simulink model "impedanceControl_ID_TUD"  (Simulink 7.9)
settings: Solver=FixedStepDiscrete  StartTime=0.0  StopTime=2000  FixedStep=Ts  RelTol=1e-3
InitFcn:
  | initialisation;
values from neighbouring files (symbols this model uses):
  A = 0*[20/180*pi;zeros(23,1);0/180*pi]    [initialisation.m]
  c = 0    [initialisation.m]
  D = diag(2*sqrt(20)*ones(1,25))    [initialisation.m]
  f = 0*1/100    (= 0)    [initialisation.m]
  P = diag(25*ones(1,25))    [initialisation.m]
  P_on = 0    [initialisation.m]
  s = 0*[10/180*pi/10;zeros(24,1)]    [initialisation.m]
  st = 0*[20/180*pi;0/180*pi;0/180*pi;0/180*pi;0/180*pi;zeros(20,1)]    [initialisation.m]
  tau_p = [torso_pitch; torso_roll; torso_yaw; left_shoulder_pitch; left_shoulder_roll; left_shoulder_yaw; left_elbow; left_wrist_prosup;      right_shoulder_pitch; right_shoulder_roll; right_shoulder_yaw; right_elbow; right_wrist_prosup; left_hip_pitch; left_hip_roll;      left_hip_yaw; left_knee; left_ankle_pitch; left_ankle_roll; right_hip_pitch;  right_hip_roll; right_hip_yaw; right_knee; right_ankle_pi ...(+22 chars)    [initialisation.m]    (also in perturbation.m)
  tin = [10;60;zeros(23,1)]    [initialisation.m]
  Tm_t = 50    [initialisation.m]    (also in perturbation.m)
  Ts = 0.1    [initialisation.m]    (also in perturbation.m)
libraries: WBCLibrary x10, commnoisgen2 x3, simulink x1
settings Model: Creator=labar  LastModifiedBy=labar

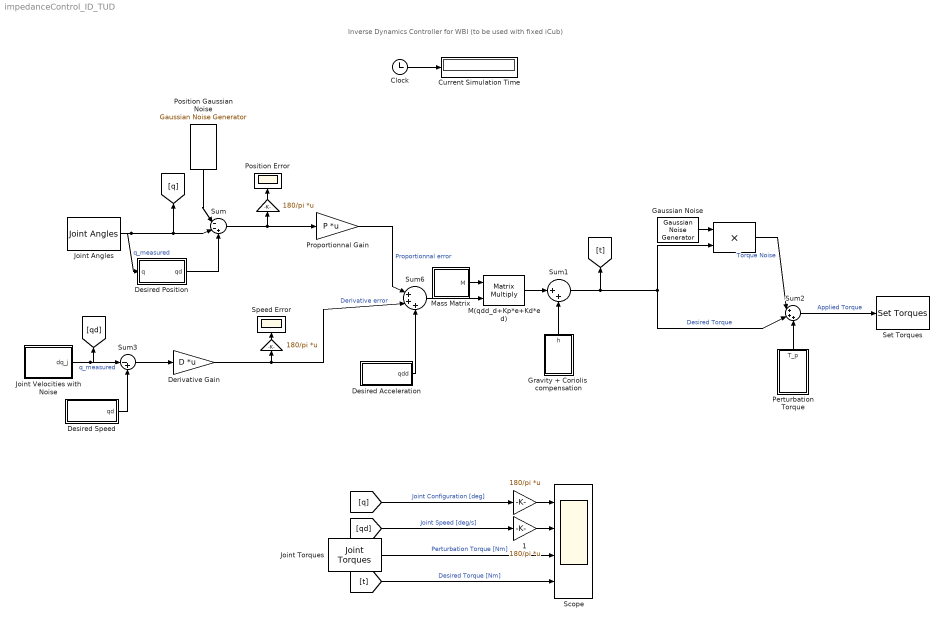
== system impedanceControl_ID_TUD ==
  note: Inverse Dynamics Controller for WBI (to be used with fixed iCub)
  "  " : Product  RndMeth=Zero
  "                  " : Gain  Gain=180/pi  Multiplication=Matrix(K*u)
  "                     " : Gain  Gain=180/pi  Multiplication=Matrix(K*u)
  "                      " : Gain  Gain=180/pi  Multiplication=Matrix(K*u)
  "                  1" : Gain  Gain=180/pi  Multiplication=Matrix(K*u)
  Clock : Clock
  Current Simulation Time : Display
  Derivative Gain : Gain  Gain=D  Multiplication=Matrix(K*u)
  Desired Acceleration : Subsystem
  Desired Position : Subsystem
  Desired Speed : Subsystem
  Gaussian Noise : commnoisgen2/Gaussian Noise Generator  m=0  d=Vt  s=41  Ts=0.1  frameBased=off  sampPerFrame=1  orient=off  outDataType=double
  Gravity + Coriolis  compensation : Subsystem
  Joint Angles : WBCLibrary/wholeBodyStates/Joint Angles  robotName=robotName  localName=localName
  Joint Torques : WBCLibrary/wholeBodyStates/Joint Torques  robotName=robotName  localName=localName
  Joint Velocities with Noise : Subsystem
  M(qdd_d+Kp*e+Kd*ed) : Product  Multiplication=Matrix(*)  RndMeth=Zero
  Mass Matrix : Subsystem
  Perturbation Torque : Subsystem
  Position Error : Scope
      settings: ShowLegends=on  SaveName=Data1
  Position Gaussian Noise : commnoisgen2/Gaussian Noise Generator  m=0  d=Vq  s=41  Ts=0.1  frameBased=off  sampPerFrame=1  orient=off  outDataType=double
  Proportionnal Gain : Gain  Gain=P  Multiplication=Matrix(K*u)
  Scope : Scope  NumInputPorts=4
      settings: ShowLegends=on  YMin=-5~-7~-5~-5  YMax=5~7~5~5  SaveName=Data
  Set Torques : WBCLibrary/wholeBodyActuators/Set Torques  val=6  robotName=robotName  localName=localName
  Speed Error : Scope
      settings: ShowLegends=on  SaveName=Data2
  Sum : Sum  Inputs=|--+
  Sum1 : Sum  Inputs=|++
  Sum2 : Sum  Inputs=|+++
  Sum3 : Sum  Inputs=|-+
  Sum6 : Sum  Inputs=|+++
  wires:
  Joint Angles/1 -> Sum/2, [q], Desired Position/1(q)  "q_measured"
  Sum1/1 -> [t], "  "/2, Sum2/2  "Desired Torque"
  Sum2/1 -> Set Torques/1  "Applied Torque"
  Clock/1 -> Current Simulation Time/1
  Proportionnal Gain/1 -> Sum6/1  "Proportionnal error"
  Derivative Gain/1 -> Sum6/2, "                      "/1  "Derivative error"
  Perturbation Torque/1(T_p) -> Sum2/3
  "  "/1 -> Sum2/1  "Torque Noise"
  Gaussian Noise/1 -> "  "/1
  Sum6/1 -> M(qdd_d+Kp*e+Kd*ed)/2
  M(qdd_d+Kp*e+Kd*ed)/1 -> Sum1/1
  Gravity + Coriolis  compensation/1(h) -> Sum1/2
  Mass Matrix/1(M) -> M(qdd_d+Kp*e+Kd*ed)/1
  Joint Velocities with Noise/1(dq_j) -> Sum3/1, [qd]  "q_measured"
  Sum3/1 -> Derivative Gain/1
  Desired Speed/1(qd) -> Sum3/2
  Desired Acceleration/1(qdd) -> Sum6/3
  Position Gaussian Noise/1 -> Sum/1
  Joint Torques/1 -> Scope/3  "Perturbation Torque [Nm]"
  [t] -> Scope/4  "Desired Torque [Nm]"
  [qd] -> "                  1"/1  "Joint Speed [deg/s]"
  "                  "/1 -> Scope/1
  [q] -> "                  "/1  "Joint Configuration [deg]"
  "                  1"/1 -> Scope/2
  "                      "/1 -> Speed Error/1
  Sum/1 -> Proportionnal Gain/1, "                     "/1
  "                     "/1 -> Position Error/1
  Desired Position/1(qd) -> Sum/3

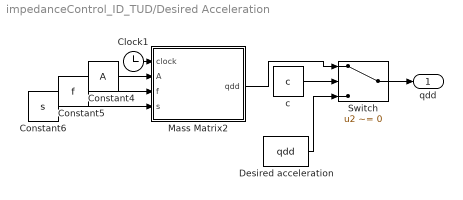
== system impedanceControl_ID_TUD/Desired Acceleration ==
  Clock1 : Clock
  Constant4 : Constant  Value=A
  Constant5 : Constant  Value=f
  Constant6 : Constant  Value=s
  Desired acceleration : FromWorkspace  VariableName=qdd  SampleTime=0
  Mass Matrix2 : MATLAB Function  TreatAsAtomicUnit=on
  Switch : Switch  Criteria=u2 ~= 0
  c : Constant  Value=c
  qdd : Outport
  wires:
  Constant4/1 -> Mass Matrix2/2(A)
  Constant5/1 -> Mass Matrix2/3(f)
  Constant6/1 -> Mass Matrix2/4(s)
  Clock1/1 -> Mass Matrix2/1(clock)
  Mass Matrix2/1(qdd) -> Switch/1
  Desired acceleration/1 -> Switch/3
  c/1 -> Switch/2
  Switch/1 -> qdd/1

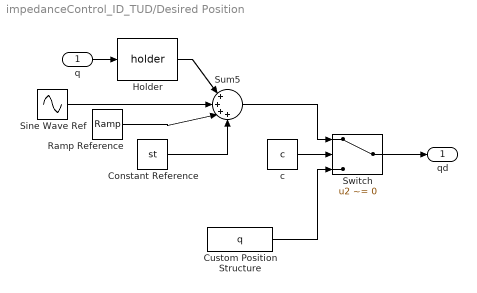
== system impedanceControl_ID_TUD/Desired Position ==
  q : Inport
  Constant Reference : Constant  Value=st
  Custom Position Structure : FromWorkspace  VariableName=q  SampleTime=0
  Holder : WBCLibrary/Utilities/holder 
  Ramp Reference : simulink/Sources/Ramp  slope=s  start=0  X0=0
  Sine Wave Ref : Sin  Amplitude=A  Frequency=f  SampleTime=0
  Sum5 : Sum  Inputs=|++++
  Switch : Switch  Criteria=u2 ~= 0
  c : Constant  Value=c
  qd : Outport
  wires:
  Holder/1 -> Sum5/1
  Sine Wave Ref/1 -> Sum5/2
  Constant Reference/1 -> Sum5/4
  Ramp Reference/1 -> Sum5/3
  q/1 -> Holder/1
  Sum5/1 -> Switch/1
  Custom Position Structure/1 -> Switch/3
  Switch/1 -> qd/1
  c/1 -> Switch/2

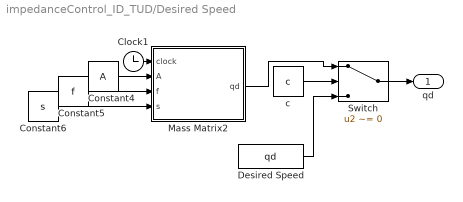
== system impedanceControl_ID_TUD/Desired Speed ==
  Clock1 : Clock
  Constant4 : Constant  Value=A
  Constant5 : Constant  Value=f
  Constant6 : Constant  Value=s
  Desired Speed : FromWorkspace  VariableName=qd  SampleTime=0
  Mass Matrix2 : MATLAB Function  TreatAsAtomicUnit=on
  Switch : Switch  Criteria=u2 ~= 0
  c : Constant  Value=c
  qd : Outport
  wires:
  Constant4/1 -> Mass Matrix2/2(A)
  Constant5/1 -> Mass Matrix2/3(f)
  Constant6/1 -> Mass Matrix2/4(s)
  Clock1/1 -> Mass Matrix2/1(clock)
  Mass Matrix2/1(qd) -> Switch/1
  Desired Speed/1 -> Switch/3
  c/1 -> Switch/2
  Switch/1 -> qd/1

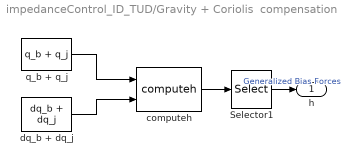
== system impedanceControl_ID_TUD/Gravity + Coriolis  compensation ==
  Selector1 : Selector  InputPortWidth=31  IndexOptions=Index vector (dialog)  Indices=[7:31]  OutputSizes=1
  computeh : WBCLibrary/wholeBodyModel/Dynamics/computeh  val=7  robotname=robotName  localname=localName
  dq_b + dq_j : WBCLibrary/wholeBodyStates/dq_b + dq_j  robotName=robotName  localName=localName  Ts=Ts
  q_b + q_j : WBCLibrary/wholeBodyStates/q_b + q_j  robotName=robotName  localName=localName  Ts=Ts
  h : Outport
  wires:
  q_b + q_j/1 -> computeh/1
  dq_b + dq_j/1 -> computeh/2
  computeh/1 -> Selector1/1
  Selector1/1 -> h/1  "Generalized Bias Forces"

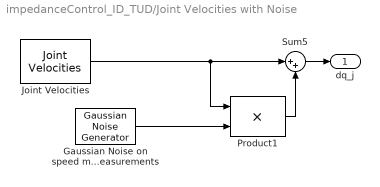
== system impedanceControl_ID_TUD/Joint Velocities with Noise ==
  Gaussian Noise on speed measurements : commnoisgen2/Gaussian Noise Generator  m=0  d=Vdq  s=41  Ts=0.1  frameBased=off  sampPerFrame=1  orient=off  outDataType=double
  Joint Velocities : WBCLibrary/wholeBodyStates/Joint Velocities  robotName=robotName  localName=localName
  Product1 : Product  RndMeth=Zero
  Sum5 : Sum  Inputs=|++
  dq_j : Outport
  wires:
  Joint Velocities/1 -> Sum5/1, Product1/1
  Gaussian Noise on speed measurements/1 -> Product1/2
  Product1/1 -> Sum5/2
  Sum5/1 -> dq_j/1

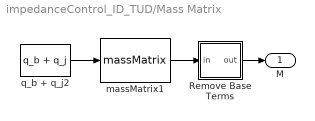
== system impedanceControl_ID_TUD/Mass Matrix ==
  Remove Base Terms : MATLAB Function  TreatAsAtomicUnit=on
  massMatrix1 : WBCLibrary/wholeBodyModel/Dynamics/massMatrix  val=8  robotname=robotName  localname=localName
  q_b + q_j2 : WBCLibrary/wholeBodyStates/q_b + q_j  robotName=robotName  localName=localName  Ts=Ts
  M : Outport
  wires:
  q_b + q_j2/1 -> massMatrix1/1
  massMatrix1/1 -> Remove Base Terms/1(in)
  Remove Base Terms/1(out) -> M/1

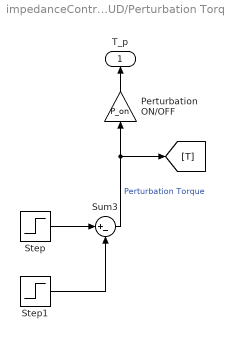
== system impedanceControl_ID_TUD/Perturbation Torque ==
  Perturbation ON/OFF : Gain  Gain=P_on
  Step : Step  Time=tin  Before=zeros(1,25)  After=tau_p  SampleTime=0
  Step1 : Step  Time=(tin+Tm_t)  Before=zeros(1,25)  After=tau_p  SampleTime=0
  Sum3 : Sum  Inputs=|+-
  T_p : Outport
  wires:
  Step1/1 -> Sum3/2
  Step/1 -> Sum3/1
  Sum3/1 -> Perturbation ON/OFF/1, [T]  "Perturbation Torque"
  Perturbation ON/OFF/1 -> T_p/1

== matlab function Desired Acceleration/Mass Matrix2 ==
  data: qdd output double; clock input double; A input double; f input double; s input double
function qdd  = fcn(clock,A,f,s)

qdd=-A.*f*f*sin(f*clock);

== matlab function Mass Matrix/Remove Base Terms ==
  data: in input double; out output double
function out = fcn(in)

out=in(7:31,7:31);

== matlab function Desired Speed/Mass Matrix2 ==
  data: qd output double; clock input double; A input double; f input double; s input double
function qd  = fcn(clock,A,f,s)

qd=A.*f*cos(f*clock)+s;
